simulink model "Exercisesimu"  (R2019a)
settings: Solver=VariableStepAuto  StartTime=0.0  StopTime=24  RelTol=1e-3
libraries: simulink_extras x1
settings Model: Creator=esthe  LastModifiedBy=esthe

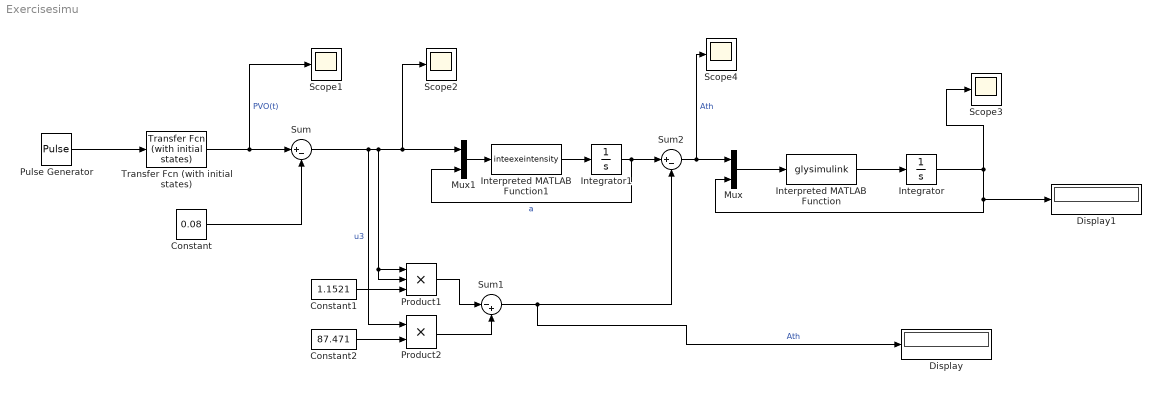
== system Exercisesimu ==
  Constant : Constant  Value=0.08
  Constant1 : Constant  Value=1.1521
  Constant2 : Constant  Value=87.471
  Display : Display
  Display1 : Display
  Integrator : Integrator
  Integrator1 : Integrator
  Interpreted MATLAB Function : MATLABFcn  MATLABFcn=glysimulink  OutputDimensions=1  Output1D=off
  Interpreted MATLAB Function1 : MATLABFcn  MATLABFcn=inteexeintensity  OutputDimensions=1  Output1D=off
  Mux : Mux  Inputs=2
  Mux1 : Mux  Inputs=2
  Product1 : Product  Inputs=3
  Product2 : Product
  Pulse Generator : DiscretePulseGenerator  PulseType=Time based  Amplitude=230  Period=24  PhaseDelay=5
  Scope{1..4} (4 alike) : Scope
  Sum : Sum  Inputs=|+-
  Sum1 : Sum  Inputs=|-+
  Sum2 : Sum  Inputs=|+-
  Transfer Fcn (with initial states) : simulink_extras/Additional Linear/Transfer Fcn (with initial states)  N=[0.8]  D="[1  0.8]"  X0=0
  wires:
  Pulse Generator/1 -> Transfer Fcn (with initial states)/1
  Transfer Fcn (with initial states)/1 -> Sum/1, Scope1/1  "PVO(t)"
  Constant/1 -> Sum/2
  Constant1/1 -> Product1/3
  Constant2/1 -> Product2/2
  Product2/1 -> Sum1/2
  Product1/1 -> Sum1/1
  Sum1/1 -> Sum2/2, Display/1  "Ath"
  Mux/1 -> Interpreted MATLAB Function/1
  Interpreted MATLAB Function/1 -> Integrator/1
  Integrator/1 -> Scope3/1, Display1/1, Mux/2
  Sum/1 -> Scope2/1, Mux1/1, Product1/2, Product1/1, Product2/1  "u3"
  Integrator1/1 -> Mux1/2, Sum2/1  "a"
  Sum2/1 -> Scope4/1, Mux/1  "Ath"
  Interpreted MATLAB Function1/1 -> Integrator1/1
  Mux1/1 -> Interpreted MATLAB Function1/1
